simulink model "vrtut2"  (R2024b)
settings: Solver=ode45  StartTime=0.0  StopTime=15  RelTol=1e-3  EnableMultiTasking=on
undefined symbols (not defined in the file or in its folder): f
libraries: instrumentlib x2
Description:
  | Simulink(R) 3D Animation(TM) - Tutorial #2
  | 
  | This model represents a tutorial example described in the documentation. See the 'Associate
  | Virtual Worlds with Simulink' chapter in the Simulink 3D Animation User's Guide.
settings Model: PacingRate=1.600000  Creator=The MathWorks, Inc.  LastModifiedBy=ethar
settings SolverCC: AlgebraicLoopSolver=TrustRegion
settings DataIOCC: LimitDataPoints=on  SaveFormat=Array  SaveOutput=off  SaveTime=off  ReturnWorkspaceOutputs=off  SignalLoggingName=logsOut
settings OptimizationCC: BlockReduction=off  BooleanDataType=off  ExpressionDepthLimit=2147483647  InitFltsAndDblsToZero=on  LifeSpan=inf
settings DebuggingCC: UnderspecifiedInitializationDetection=Classic  MergeDetectMultiDrivingBlocksExec=none  CheckExecutionContextPreStartOutputMsg=on  SignalResolutionControl=TryResolveAllWithWarning  MultiTaskDSMMsg=warning  MultiTaskCondExecSysMsg=none  FcnCallInpInsideContextMsg=warning  UnconnectedInputMsg=warning  UnconnectedOutputMsg=warning  UnconnectedLineMsg=warning  StateNameClashWarn=warning  SymbolicDimsDataTypeCodeGenerationDiagnostic=none  SFUnexpectedBacktrackingDiag=warning  SFNoUnconditionalDefaultTransitionDiag=warning  SFExecutionAtInitializationDiag=none  ArithmeticOperatorsInVariantConditions=warning
settings HardwareCC: ProdBitPerPointer=32  ProdBitPerSizeT=32  ProdBitPerPtrDiffT=32  ProdLargestAtomicFloat=None  ProdIntDivRoundTo=Undefined  ProdEndianess=Unspecified  ProdWordSize=32  ProdHWDeviceType=32-bit Generic  TargetUnknown=on
settings ModelReferenceCC: UpdateModelReferenceTargets=IfOutOfDate  EnableRefExpFcnMdlSchedulingChecks=on  PropagateSignalLabelsOutOfModel=off
settings SFSimCC: SimUseLocalCustomCode=off  CustomCodeUndefinedFunction=UseInterfaceOnly
settings RTWCC: RTWUseLocalCustomCode=off  GPUComputeCapability=3.5
settings CodeAppCC: StateflowObjectComments=on
settings GRTTargetCC: TargetFcnLib=ansi_tfl_tmw.mat  TargetLangStandard=C89/C90 (ANSI)  CombineOutputUpdateFcns=off  GRTInterface=on
settings ConfigComp: CovMetricSettings=d  CovSaveCumulativeToWorkspaceVar=on  CovSaveSingleToWorkspaceVar=on  CovExternalEMLEnable=off  CovSFcnEnable=off

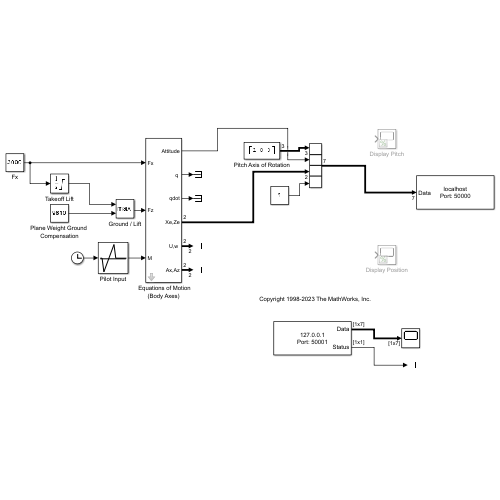
[thumbnail: Simulink's stored preview of the top-level diagram]
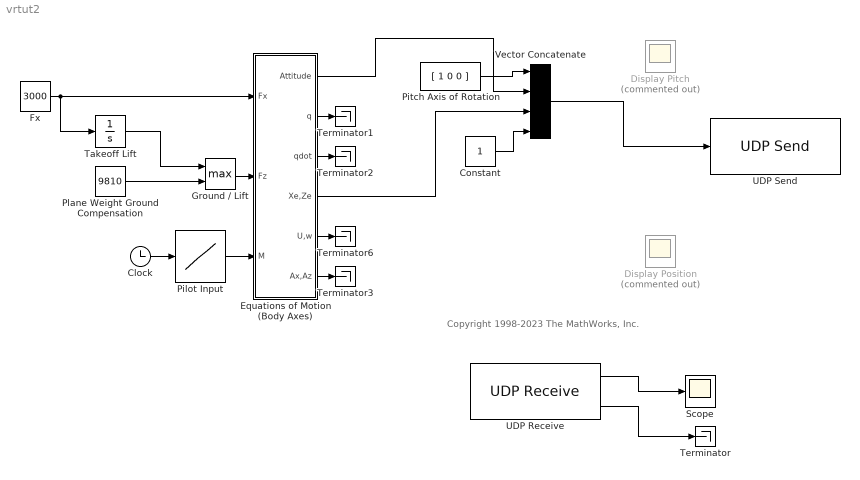
== system vrtut2 ==
  note: Copyright 1998-2023 The MathWorks, Inc.
  " Equations of Motion (Body Axes)" : Subsystem  mask(3 DOF equations of motion){v_ini=0, theta_ini=0, alpha_ini=0, q_ini=0, pos_ini=[0 0], mass=1000, Iyy=1000, g=-9.81}
      mask prompts: v_ini "Initial velocity [m/s]:"; theta_ini "Initial body attitude [rad]:"; alpha_ini "Initial incidence [rad]:"; q_ini "Initial body rotation rate [rad/sec]:"; pos_ini "Initial position (x z) [m]:"; mass "Mass [Kg]:"; Iyy "Inertia [Kg.m^2]:"; g "Acceleration due to gravity [m/s/s]:"
      mask help: Integrates the 3 degrees of freedom equations of motion to determine body position, velocity, attitude and related values.
      mask init:
      | U0 = v_ini*cos(alpha_ini);
      | w0 = v_ini*sin(alpha_ini);
      settings: LibrarySourceBlock=|
      | aerospace/3DoF
      | Equations
      | of
      | Motion / Equations of Motion
      | (Body Axes)
      mask Help:
      | <p>This block models the 3 degrees of freedom equations of motion to determine body position, velocity, attitude and other related values.</p>
      | 
      | <p>A 3-down configuration for the body coordinates ( X axis pointing toward nose of body, and  Z axis pointing towards earth) is used in this block.</p>
      | 
      | <p>Gravitational force on the body is already accounted for in this block.</p>
      | 
      | <p>Some block outputs contain more than one signal as described below.</p>
      | 
      | <p><H4>Block  Inputs</H4>
      | <ul>
      |     <li>Forces on the body in X direction - Fx ( N )</li>
      |     <li>Forces on the body in Z direction - Fz ( N ) </li>
      |     <li>Moments on the body along Y direction - M ( N-m )</li>
      | </ul>
      | </p>
      | <p><H4>Block Outputs</H4>
      | <ul>
      |     <li>Pitch angle - Attitude ( radians )</li>
      |     <li>Pitch rate - q ( radians/sec )</li>
      |     <li>Pitch acceleration - qdot ( radians/sec^2 )</li>
      | </ul>
      | </p>
      | <p><H4>Block Vector Output - Xe, Ze </H4>
      | <ul>
      |     <li>Position in X direction in Earth coordinates - Xe ( m )</li>
      |     <li>Position in Z direction in Earth coordinates - Ze ( m )</li>
      | </ul>
      | </p>
      | <p><H4>Block Vector Output - U,w </H4>
      | <ul>
      |     <li>Translational velocity in X direction - U ( m/sec )</li>
      |     <li>Translational velocity in Z direction - w ( m/sec )</li>
      | </ul>
      | </p>
      | <p><H4>Block Vector Output - Ax, Az </H4>
      | <ul>
      |     <li>Acceleration in X direction due to body forces - Ax ( m/sec^2 )</li>
      |     <li>Acceleration in Z direction due to body forces - Az ( m/sec^2 )</li>
      | </ul>
      | </p>
  Clock : Clock
  Constant : Constant
  Display Pitch : Scope  Commented=on
  Display Position : Scope  Commented=on
  Fx : Constant  Value=3000
  Ground / Lift : MinMax  Function=max  Inputs=2  InputSameDT=on  SaturateOnIntegerOverflow=on
  Pilot Input : Lookup  InputValues=[0 1 2 8 9 15]  Table=[0 0 -20 20 0 0]
  Pitch Axis of Rotation : Constant  Value=[ 1 0 0 ]
  Plane Weight Ground Compensation : Constant  Value=9810
  Scope : Scope
  Takeoff Lift : Integrator  LimitOutput=on  UpperSaturationLimit=11000  LowerSaturationLimit=-Inf
  Terminator{,1..3,6} (5 alike) : Terminator
  UDP Receive : instrumentlib/UDP Receive  LocalAddress=127.0.0.1  LocalPort=50001  EnablePortSharing=off  Host=localhost  Port=65343  GetLatestData=on  DataSize=[ 1, 7 ]  DataType=double  ASCIIFormatting=%f,  Terminator=LF  CustomTerminator=10  ByteOrder=big-endian  EnableBlockingMode=off  Timeout=10  SampleTime=0.01  SimulateUsing=Interpreted execution
  UDP Send : instrumentlib/UDP Send  Host=localhost  Port=50000  LocalAddress=127.0.0.1  LocalPort=-1  EnablePortSharing=on  OutputDatagramPacketSize=512  ByteOrder=big-endian  EnableBlockingMode=on  SimulateUsing=Interpreted execution
  Vector Concatenate : Concatenate  NumInputs=4
  wires:
  Pitch Axis of Rotation/1 -> Vector Concatenate/1
  " Equations of Motion (Body Axes)"/1(Attitude) -> Vector Concatenate/2
  " Equations of Motion (Body Axes)"/2("q ") -> Terminator1/1
  " Equations of Motion (Body Axes)"/3(qdot) -> Terminator2/1
  Ground / Lift/1 -> " Equations of Motion (Body Axes)"/2(Fz)
  Takeoff Lift/1 -> Ground / Lift/1
  Plane Weight Ground Compensation/1 -> Ground / Lift/2
  Clock/1 -> Pilot Input/1
  Pilot Input/1 -> " Equations of Motion (Body Axes)"/3(M)
  Fx/1 -> " Equations of Motion (Body Axes)"/1(Fx), Takeoff Lift/1
  " Equations of Motion (Body Axes)"/4(Xe,Ze) -> Vector Concatenate/3
  Vector Concatenate/1 -> UDP Send/1
  " Equations of Motion (Body Axes)"/6(Ax,Az) -> Terminator3/1
  " Equations of Motion (Body Axes)"/5("U,w ") -> Terminator6/1
  Constant/1 -> Vector Concatenate/4
  UDP Receive/1 -> Scope/1
  UDP Receive/2 -> Terminator/1

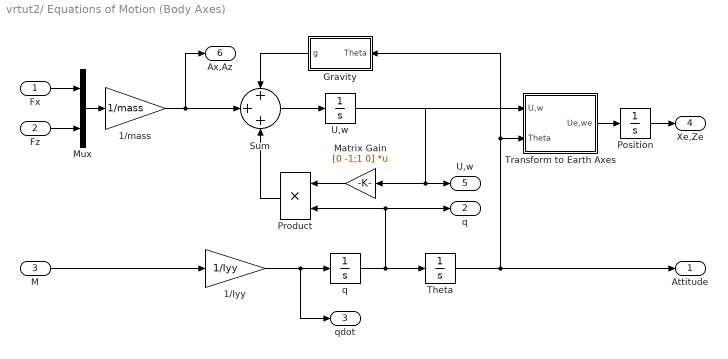
== system vrtut2/ Equations of Motion (Body Axes) ==
  Fx : Inport
  Fz : Inport  Port=2
  M : Inport  Port=3
  1/Iyy : Gain  Gain=1/Iyy  SaturateOnIntegerOverflow=on  OutDataTypeStr=Inherit: Same as input  ParamDataTypeStr=Inherit: Same as input
  1/mass : Gain  Gain=1/mass  SaturateOnIntegerOverflow=on  OutDataTypeStr=Inherit: Same as input  ParamDataTypeStr=Inherit: Same as input
  Gravity : Subsystem
  Matrix Gain : Gain  Gain=[0 -1;1 0]  Multiplication=Matrix(K*u)  SaturateOnIntegerOverflow=on  OutDataTypeStr=Inherit: Same as input  ParamDataTypeStr=Inherit: Same as input
  Mux : Mux  Inputs=2
  Position : Integrator  InitialCondition=pos_ini
  Product : Product  InputSameDT=on  RndMeth=Zero  SaturateOnIntegerOverflow=on  OutDataTypeStr=Inherit: Same as first input
  Sum : Sum  Inputs=+++  InputSameDT=on  SaturateOnIntegerOverflow=on  OutDataTypeStr=Inherit: Same as first input
  Theta : Integrator  InitialCondition=theta_ini
  Transform to Earth Axes : Subsystem
  U,w : Integrator  InitialCondition=[U0 w0]
  q : Integrator  InitialCondition=q_ini
  Attitude : Outport  InitialOutput=0  VectorParamsAs1DForOutWhenUnconnected=off
  "q " : Outport  Port=2  InitialOutput=0  VectorParamsAs1DForOutWhenUnconnected=off
  qdot : Outport  Port=3  InitialOutput=0  VectorParamsAs1DForOutWhenUnconnected=off
  Xe,Ze : Outport  Port=4  InitialOutput=0  VectorParamsAs1DForOutWhenUnconnected=off
  "U,w " : Outport  Port=5  InitialOutput=0  VectorParamsAs1DForOutWhenUnconnected=off
  Ax,Az : Outport  Port=6  InitialOutput=0  VectorParamsAs1DForOutWhenUnconnected=off
  wires:
  Gravity/1(g) -> Sum/1
  1/mass/1 -> Sum/2, Ax,Az/1
  Product/1 -> Sum/3
  Mux/1 -> 1/mass/1
  Fz/1 -> Mux/2
  Fx/1 -> Mux/1
  Transform to Earth Axes/1(Ue,we) -> Position/1
  Matrix Gain/1 -> Product/1
  Position/1 -> Xe,Ze/1
  U,w/1 -> "U,w "/1, Transform to Earth Axes/1(U,w), Matrix Gain/1
  Theta/1 -> Gravity/1(Theta), Transform to Earth Axes/2(Theta), Attitude/1
  1/Iyy/1 -> qdot/1, q/1
  M/1 -> 1/Iyy/1
  q/1 -> Product/2, "q "/1, Theta/1
  Sum/1 -> U,w/1

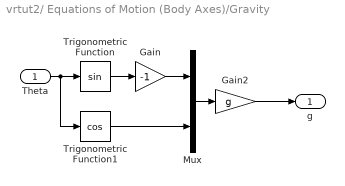
== system vrtut2/ Equations of Motion (Body Axes)/Gravity ==
  Theta : Inport
  Gain : Gain  Gain=-1  SaturateOnIntegerOverflow=on  OutDataTypeStr=Inherit: Same as input  ParamDataTypeStr=Inherit: Same as input
  Gain2 : Gain  Gain=g  SaturateOnIntegerOverflow=on  OutDataTypeStr=Inherit: Same as input  ParamDataTypeStr=Inherit: Same as input
  Mux : Mux  Inputs=2
  Trigonometric Function : Trigonometry
  Trigonometric Function1 : Trigonometry  Operator=cos
  g : Outport  VectorParamsAs1DForOutWhenUnconnected=off
  wires:
  Gain2/1 -> g/1
  Mux/1 -> Gain2/1
  Trigonometric Function1/1 -> Mux/2
  Gain/1 -> Mux/1
  Trigonometric Function/1 -> Gain/1
  Theta/1 -> Trigonometric Function/1, Trigonometric Function1/1

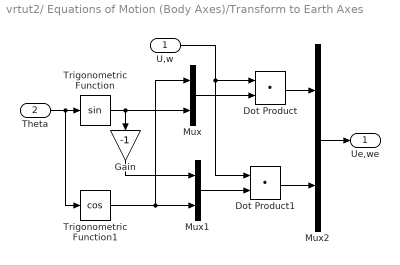
== system vrtut2/ Equations of Motion (Body Axes)/Transform to Earth Axes ==
  U,w : Inport
  Theta : Inport  Port=2
  Dot Product : DotProduct  OutDataTypeStr=Inherit: Inherit via internal rule
  Dot Product1 : DotProduct  OutDataTypeStr=Inherit: Inherit via internal rule
  Gain : Gain  Gain=-1  SaturateOnIntegerOverflow=on  OutDataTypeStr=Inherit: Same as input  ParamDataTypeStr=Inherit: Same as input
  Mux : Mux  Inputs=2
  Mux1 : Mux  Inputs=2
  Mux2 : Mux  Inputs=2
  Trigonometric Function : Trigonometry
  Trigonometric Function1 : Trigonometry  Operator=cos
  Ue,we : Outport  VectorParamsAs1DForOutWhenUnconnected=off
  wires:
  Gain/1 -> Mux1/1
  Trigonometric Function/1 -> Mux/2, Gain/1
  Theta/1 -> Trigonometric Function1/1, Trigonometric Function/1
  U,w/1 -> Dot Product1/1, Dot Product/1
  Mux/1 -> Dot Product/2
  Mux2/1 -> Ue,we/1
  Dot Product1/1 -> Mux2/2
  Dot Product/1 -> Mux2/1
  Mux1/1 -> Dot Product1/2
  Trigonometric Function1/1 -> Mux1/2, Mux/1
